simulink model "checkData"  (Simulink 7.1)
settings: Solver=FixedStepDiscrete  StartTime=0.0  StopTime=10.0  FixedStep=0.05  RelTol=1e-3
settings Model: Creator=jrivitus  LastModifiedBy=jrivitus

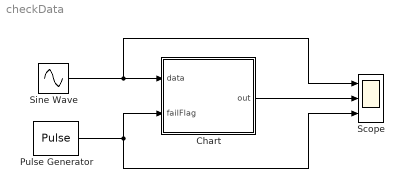
== system checkData ==
  Chart : Stateflow chart
  Pulse Generator : DiscretePulseGenerator  Period=30  SampleTime=0.05
  Scope : Scope  NumInputPorts=3
      settings: YMin=-5~-5~-5  YMax=5~5~5
  Sine Wave : Sin  SampleTime=0.05
  wires:
  Chart/1(out) -> Scope/2
  Sine Wave/1 -> Scope/1, Chart/1(data)
  Pulse Generator/1 -> Scope/3, Chart/2(failFlag)

== stateflow chart Chart ==
  (default) -> (junction 3)
  (junction 3) -> (junction 4) [order 1] : [failFlag == 1]
  (junction 4) -> (junction 13) : {
      | count = 1;
      | }
  (junction 5) -> (junction 6) [order 1] : [count == 5]
  (junction 5) -> (junction 7) [order 2] : {count = count + 1;}
  (junction 6) -> (junction 8) : {count = 0;}
  (junction 8) -> (junction 7)
  (junction 3) -> (junction 11) [order 2]
  (junction 9) -> (junction 12) [order 2] : {out = data;}
  (junction 9) -> (junction 10) [order 1] : [count > 0]
  (junction 10) -> (junction 5) : {out = 0;}
  (junction 7) -> (junction 12)
  (junction 11) -> (junction 9)
  (junction 13) -> (junction 11)
  data: count local double; data input double; failFlag input double; out output double
